simulink model "task2"  (R2024a)
settings: Solver=VariableStepAuto  StartTime=0.0  StopTime=10.0  MaxStep=0.01  RelTol=1e-3
undefined symbols (not defined in the file): Abar, Bbar, Cbar, D, Gamma, Gamma_g, invQ, K, Kf, Kg, L, wg0, wg_bar0, xf0, xf_hat0, Y, Yg
settings Model: Creator=sizgr  LastModifiedBy=sizgr

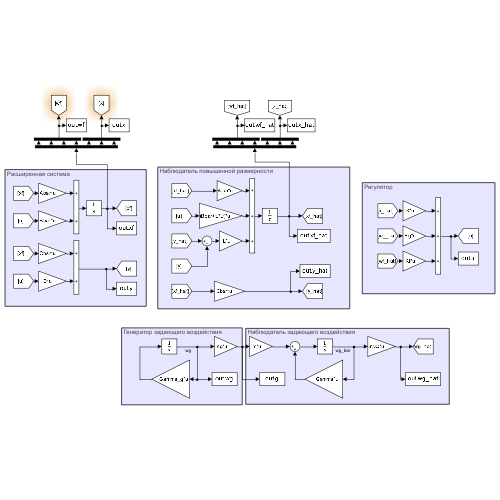
[thumbnail: Simulink's stored preview of the top-level diagram]
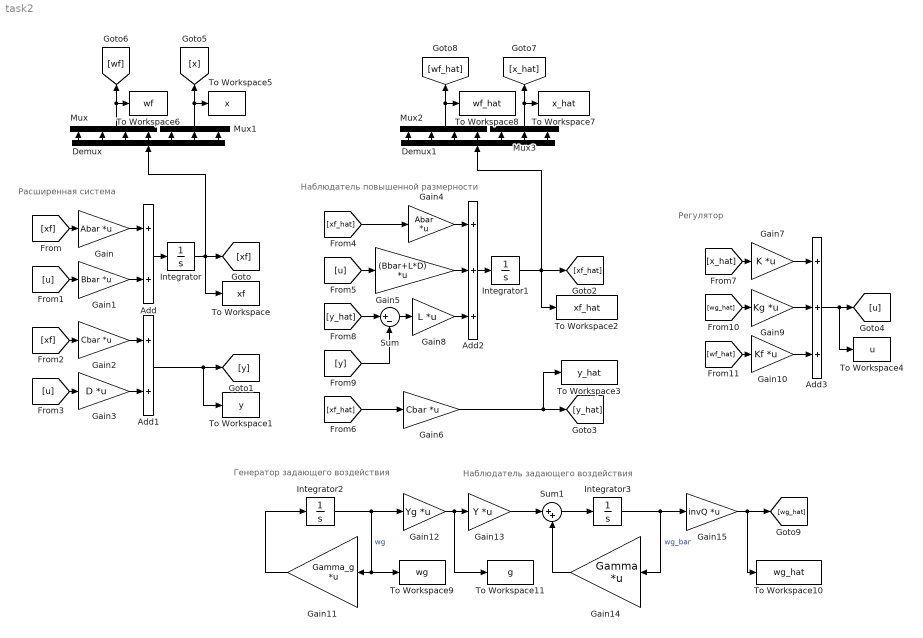
== system task2 ==
  note: Генератор задающего воздействия
  note: Наблюдатель задающего воздействия
  note: Регулятор
  note: Расширенная система
  note: Наблюдатель повышенной размерности
  Add : Sum
  Add1 : Sum
  Add2 : Sum  Inputs=+++
  Add3 : Sum  Inputs=+++
  Demux : Demux  Outputs=7
  Demux1 : Demux  Outputs=7
  Gain : Gain  Gain=Abar  Multiplication=Matrix(K*u)
  Gain1 : Gain  Gain=Bbar  Multiplication=Matrix(K*u)
  Gain10 : Gain  Gain=Kf  Multiplication=Matrix(K*u)
  Gain11 : Gain  Gain=Gamma_g  Multiplication=Matrix(K*u)
  Gain12 : Gain  Gain=Yg  Multiplication=Matrix(K*u)
  Gain13 : Gain  Gain=Y  Multiplication=Matrix(K*u)
  Gain14 : Gain  Gain=Gamma  Multiplication=Matrix(K*u)
  Gain15 : Gain  Gain=invQ  Multiplication=Matrix(K*u)
  Gain2 : Gain  Gain=Cbar  Multiplication=Matrix(K*u)
  Gain3 : Gain  Gain=D  Multiplication=Matrix(K*u)
  Gain4 : Gain  Gain=Abar  Multiplication=Matrix(K*u)
  Gain5 : Gain  Gain=(Bbar+L*D)  Multiplication=Matrix(K*u)
  Gain6 : Gain  Gain=Cbar  Multiplication=Matrix(K*u)
  Gain7 : Gain  Gain=K  Multiplication=Matrix(K*u)
  Gain8 : Gain  Gain=L  Multiplication=Matrix(K*u)
  Gain9 : Gain  Gain=Kg  Multiplication=Matrix(K*u)
  Integrator : Integrator  InitialCondition=xf0
  Integrator1 : Integrator  InitialCondition=xf_hat0
  Integrator2 : Integrator  InitialCondition=wg0
  Integrator3 : Integrator  InitialCondition=wg_bar0
  Mux : Mux
  Mux1 : Mux  Inputs=3
  Mux2 : Mux
  Mux3 : Mux  Inputs=3
  Sum : Sum  Inputs=|+-
  Sum1 : Sum  Inputs=|++
  To Workspace : ToWorkspace  VariableName=xf  SaveFormat=Timeseries  SampleTime=-1
  To Workspace1 : ToWorkspace  VariableName=y  SaveFormat=Timeseries  SampleTime=-1
  To Workspace10 : ToWorkspace  VariableName=wg_hat  SaveFormat=Timeseries  SampleTime=-1
  To Workspace11 : ToWorkspace  VariableName=g  SaveFormat=Timeseries  SampleTime=-1
  To Workspace2 : ToWorkspace  VariableName=xf_hat  SaveFormat=Timeseries  SampleTime=-1
  To Workspace3 : ToWorkspace  VariableName=y_hat  SaveFormat=Timeseries  SampleTime=-1
  To Workspace4 : ToWorkspace  VariableName=u  SaveFormat=Timeseries  SampleTime=-1
  To Workspace5 : ToWorkspace  VariableName=x  SaveFormat=Timeseries  SampleTime=-1
  To Workspace6 : ToWorkspace  VariableName=wf  SaveFormat=Timeseries  SampleTime=-1
  To Workspace7 : ToWorkspace  VariableName=x_hat  SaveFormat=Timeseries  SampleTime=-1
  To Workspace8 : ToWorkspace  VariableName=wf_hat  SaveFormat=Timeseries  SampleTime=-1
  To Workspace9 : ToWorkspace  VariableName=wg  SaveFormat=Timeseries  SampleTime=-1
  wires:
  Add/1 -> Integrator/1
  Gain/1 -> Add/1
  Gain1/1 -> Add/2
  Integrator/1 -> Demux/1, To Workspace/1, [xf]
  [xf] -> Gain/1
  [u] -> Gain1/1
  Gain2/1 -> Add1/1
  [u] -> Gain3/1
  Add1/1 -> [y], To Workspace1/1
  [xf] -> Gain2/1
  Gain3/1 -> Add1/2
  Gain6/1 -> To Workspace3/1, [y_hat]
  [u] -> Gain5/1
  Add2/1 -> Integrator1/1
  Gain4/1 -> Add2/1
  [xf_hat] -> Gain4/1
  [xf_hat] -> Gain6/1
  Gain5/1 -> Add2/2
  Gain8/1 -> Add2/3
  Sum/1 -> Gain8/1
  [y_hat] -> Sum/1
  [y] -> Sum/2
  Add3/1 -> To Workspace4/1, [u]
  Gain7/1 -> Add3/1
  Gain9/1 -> Add3/2
  Gain10/1 -> Add3/3
  [x_hat] -> Gain7/1
  [wg_hat] -> Gain9/1
  [wf_hat] -> Gain10/1
  Demux/1 -> Mux/1
  Demux/2 -> Mux/2
  Demux/3 -> Mux/3
  Demux/4 -> Mux/4
  Demux/5 -> Mux1/1
  Demux/6 -> Mux1/2
  Demux/7 -> Mux1/3
  Mux/1 -> [wf], To Workspace6/1
  Mux1/1 -> To Workspace5/1, [x]
  Demux1/5 -> Mux3/1
  Integrator1/1 -> Demux1/1, To Workspace2/1, [xf_hat]
  Demux1/4 -> Mux2/4
  Demux1/1 -> Mux2/1
  Demux1/2 -> Mux2/2
  Demux1/7 -> Mux3/3
  Demux1/3 -> Mux2/3
  Mux3/1 -> To Workspace7/1, [x_hat]
  Demux1/6 -> Mux3/2
  Mux2/1 -> [wf_hat], To Workspace8/1
  Integrator2/1 -> Gain12/1, To Workspace9/1, Gain11/1  "wg"
  Gain11/1 -> Integrator2/1
  Gain12/1 -> To Workspace11/1, Gain13/1
  Gain13/1 -> Sum1/1
  Sum1/1 -> Integrator3/1
  Integrator3/1 -> Gain15/1, Gain14/1  "wg_bar"
  Gain14/1 -> Sum1/2
  Gain15/1 -> To Workspace10/1, [wg_hat]
